simulink model "ffpid_ctrl"  (R2016a)
settings: Solver=ode5  StartTime=0.0  StopTime=inf  FixedStep=0.01  RelTol=1e-3
undefined symbols (not defined in the file or in its folder): Humusoft, MF644, robot
libraries: sldrtlib x2
settings Model: Creator=julianleland  LastModifiedBy=julianleland
settings HardwareCC: ProdBitPerLong=64  ProdLargestAtomicFloat=None  ProdHWDeviceType=Intel->x86-64  TargetBitPerLong=64  TargetBitPerPointer=64  TargetIntDivRoundTo=Zero  TargetEndianess=LittleEndian  TargetWordSize=64  TargetHWDeviceType=Intel->x86-64
settings RTWCC: SystemTargetFile=sldrt.tlc  TemplateMakefile=sldrt.tmf  Description=Simulink Desktop Real-Time  RTWCompilerOptimization=on
settings CodeAppCC: MaxIdLength=95
settings SimulinkDesktopRealTimeCC: TargetPreCompLibLocation=/Applications/MATLAB_R2016a.app/toolbox/sldrt/lib/maci64  TargetLangStandard=C89/C90 (ANSI)  SupportVariableSizeSignals=off

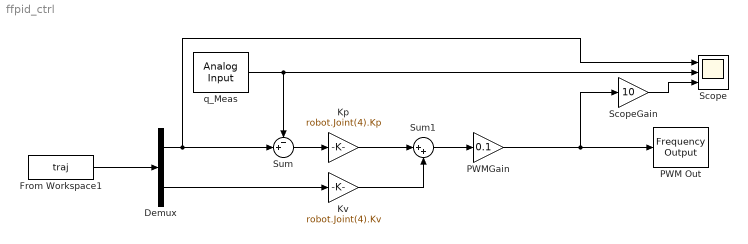
== system ffpid_ctrl ==
  Demux : Demux  Outputs=2
  From Workspace1 : FromWorkspace  VariableName=traj  Interpolate=off  OutputAfterFinalValue=Setting to zero
  Kp : Gain  Gain=robot.Joint(4).Kp
  Kv : Gain  Gain=robot.Joint(4).Kv
  PWM Out : sldrtlib/Frequency Output  SampleTime=-1  MaxMissedTicks=10  ShowMissedTicks=off  YieldWhenWaiting=off  DrvName=Humusoft/MF644  DrvAddress=4294967295  DrvOptions=585  Channels=4  FrequencySource=1  Frequency=10  FrequencyFinalValue=[]  DutySource=2  Duty=0.5  DutyFinalValue=0.5
      settings: AttributesFormatString=Humusoft\nMF644 [auto]
  PWMGain : Gain  Gain=0.1
  Scope : Scope  NumInputPorts=3
  ScopeGain : Gain  Gain=10
  Sum : Sum  Inputs=-+|
  Sum1 : Sum  Inputs=|++
  q_Meas : sldrtlib/Analog Input  SampleTime=-1  MaxMissedTicks=10  ShowMissedTicks=off  YieldWhenWaiting=off  DrvName=Humusoft/MF644  DrvAddress=4294967295  DrvOptions=585  Channels=5  RangeMode=1  VoltRange=1  DataType=1
      settings: AttributesFormatString=Humusoft\nMF644 [auto]
  wires:
  q_Meas/1 -> Scope/2, Sum/1
  From Workspace1/1 -> Demux/1
  Demux/1 -> Scope/1, Sum/2
  Demux/2 -> Kv/1
  Sum/1 -> Kp/1
  Sum1/1 -> PWMGain/1
  Kv/1 -> Sum1/2
  Kp/1 -> Sum1/1
  PWMGain/1 -> ScopeGain/1, PWM Out/1
  ScopeGain/1 -> Scope/3
